simulink model "templateFromStructSimulinkS"  (R2018b)
settings: Solver=VariableStepAuto  StartTime=0.0  StopTime=10.0  RelTol=1e-3
values from neighbouring files (symbols this model uses):
  A = rand(3,2)    [templateFromFile.m]    (also in templateFromStruct.m; templateFromStructSimulink.m; templateFromStructSimulink_dylib.m; templateFromStruct_dylib.m)
  B = rand(2,4)    [templateFromFile.m]    (also in templateFromStruct.m; templateFromStructSimulink.m; templateFromStructSimulink_dylib.m; templateFromStruct_dylib.m)
  C = rand(3,4)    [templateFromFile.m]    (also in templateFromStruct.m; templateFromStructSimulink.m; templateFromStructSimulink_dylib.m; templateFromStruct_dylib.m)
settings Model: Creator=hespanha  LastModifiedBy=hespanha

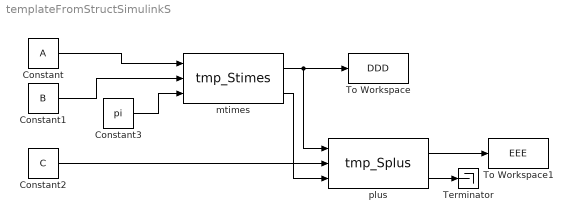
== system templateFromStructSimulinkS ==
  Constant : Constant  Value=A
  Constant1 : Constant  Value=B
  Constant2 : Constant  Value=C
  Constant3 : Constant  Value=pi
  Terminator : Terminator
  To Workspace : ToWorkspace  VariableName=DDD  SampleTime=-1
  To Workspace1 : ToWorkspace  VariableName=EEE  SampleTime=-1
  mtimes : S-Function  FunctionName=tmp_Stimes  SFunctionDeploymentMode=off  EnableBusSupport=off
  plus : S-Function  FunctionName=tmp_Splus  SFunctionDeploymentMode=off  EnableBusSupport=off
  wires:
  Constant/1 -> mtimes/1
  mtimes/1 -> plus/1, To Workspace/1
  plus/1 -> To Workspace1/1
  Constant1/1 -> mtimes/2
  Constant2/1 -> plus/2
  mtimes/2 -> plus/3
  plus/2 -> Terminator/1
  Constant3/1 -> mtimes/3
